simulink model "altitude_contr"  (R2024a)
settings: Solver=FixedStepAuto  StartTime=0.0  StopTime=300  FixedStep=sample_time  RelTol=1e-3
undefined symbols (not defined in the file): A, B, C, D
libraries: slpidlib x1
settings Model: Creator=Lorenzo-Desk  LastModifiedBy=Lorenzo-Desk
settings DataIOCC: ExternalInput=[t,u]

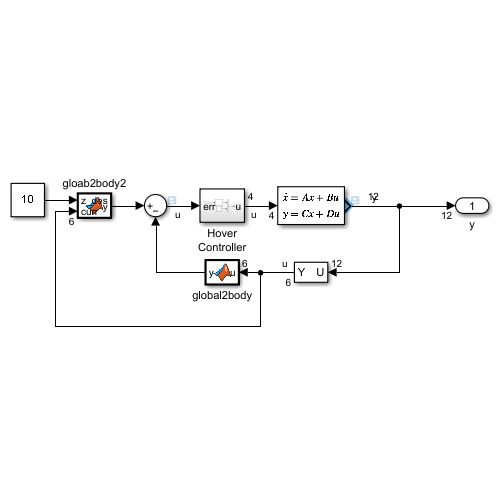
[thumbnail: Simulink's stored preview of the top-level diagram]
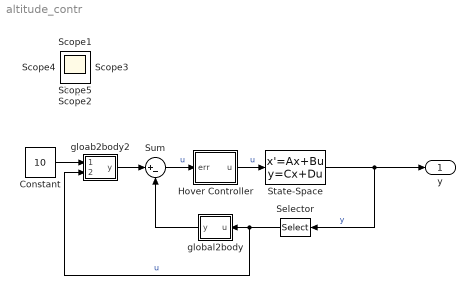
== system altitude_contr ==
  Constant : Constant  Value=10
  Hover Controller : Subsystem
  Selector : Selector  InputPortWidth=12  IndexOptions=Index vector (dialog)  Indices=[1 2 3 7 8 9]  OutputSizes=1
  State-Space : StateSpace  A=A  B=B  C=C  D=D  InitialCondition=0
  Sum : Sum  Inputs=|+-
  gloab2body2 : MATLAB Function  TreatAsAtomicUnit=on
  global2body : MATLAB Function  TreatAsAtomicUnit=on
  y : Outport
  Scope{,1..5} (6 alike) : Scope
  wires:
  State-Space/1 -> Selector/1, y/1  "y"
  Sum/1 -> Hover Controller/1(err)  "u"
  Selector/1 -> gloab2body2/2(curr), global2body/1(u)  "u"
  Constant/1 -> gloab2body2/1(z_des)
  Hover Controller/1(u) -> State-Space/1  "u"
  global2body/1(y) -> Sum/2
  gloab2body2/1(y) -> Sum/1

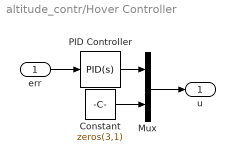
== system altitude_contr/Hover Controller ==
  err : Inport
  Constant : Constant  Value=zeros(3,1)
  Mux : Mux  Inputs=2
  PID Controller : slpidlib/PID Controller  Controller=PID  Form=Parallel  TimeDomain=Continuous-time  UseExternalTs=off  SampleTime=-1  IntegratorMethod=Forward Euler  FilterMethod=Forward Euler  ControllerParametersSource=internal  P=-0.00282534654260682  I=-0.31298101277526e-06  UseKiTs=off  D=-0.14108397495746  UseExternalDerivativeSource=off  N=25.5263564368939  UseFilter=on  TunerSelectOption=Transfer Function Based (PID Tuner App)  InitialConditionSource=internal  InitialConditionForIntegrator=0  InitialConditionForFilter=0  DifferentiatorICPrevScaledInput=0  ExternalReset=none  TrackingMode=off  Kt=1  LimitOutput=on  SatLimitsSource=internal  UpperSaturationLimit=18  LowerSaturationLimit=-18  LinearizeAsGain=on  AntiWindupMode=clamping  Kb=1  LimitIntegrator=on  UpperIntegratorSaturationLimit=20  LowerIntegratorSaturationLimit=-20  POutMin=[]  POutMax=[]  IOutMin=[]  IOutMax=[]  DOutMin=[]  DOutMax=[]  NOutMin=[]  NOutMax=[]  SumOutMin=[]  SumOutMax=[]  SaturationOutMin=[]  SaturationOutMax=[]  PParamMin=[]  PParamMax=[]  IParamMin=[]  IParamMax=[]  DParamMin=[]  DParamMax=[]  NParamMin=[]  NParamMax=[]  KbParamMin=[]  KbParamMax=[]  KtParamMin=[]  KtParamMax=[]  KbOutMin=[]  KbOutMax=[]  KtOutMin=[]  KtOutMax=[]  IntegratorOutMin=[]  IntegratorOutMax=[]  FilterOutMin=[]  FilterOutMax=[]  SumI1OutMin=[]  SumI1OutMax=[]  SumI2OutMin=[]  SumI2OutMax=[]  SumI3OutMin=[]  SumI3OutMax=[]  SumI4OutMin=[]  SumI4OutMax=[]  SumDOutMin=[]  SumDOutMax=[]  DifferentiatorOutMin=[]  DifferentiatorOutMax=[]  FilterDiffOutCoefMin=[]  FilterDiffOutCoefMax=[]  ReciprocalOutMin=[]  ReciprocalOutMax=[]  SumDenOutMin=[]  SumDenOutMax=[]  SumNumOutMin=[]  SumNumOutMax=[]  DivideOutMin=[]  DivideOutMax=[]  UdiffTsProdOutMin=[]  UdiffTsProdOutMax=[]  NTsProdOutMin=[]  NTsProdOutMax=[]  UintegralTsProdOutMin=[]  UintegralTsProdOutMax=[]  UngainTsProdOutMin=[]  UngainTsProdOutMax=[]  ClampingZeroOutDataTypeStr=Inherit: Inherit via back propagation  ClampingZeroOutMin=[]  ClampingZeroOutMax=[]  FilterDenConstantOutDataTypeStr=Inherit: Inherit via back propagation  FilterDenConstantOutMin=[]  FilterDenConstantOutMax=[]  PCopyOutDataTypeStr=Inherit: Inherit via back propagation  PCopyOutMin=[]  PCopyOutMax=[]  NCopyOutDataTypeStr=Inherit: Inherit via back propagation  NCopyOutMin=[]  NCopyOutMax=[]  IntegratorContinuousStateAttributes=''  IntegratorStateMustResolveToSignalObject=off  IntegratorRTWStateStorageClass=Auto  FilterContinuousStateAttributes=''  FilterStateMustResolveToSignalObject=off  FilterRTWStateStorageClass=Auto  ParallelPVariant=InternalParameters  IdealPVariant=Disabled  IVariant=InternalParameters  DVariant=InternalParameters  IntegratorVariant=Continuous  SatVariant=Enabled  AWVariant=ContClampingParallel  PCopyVariant=Disabled  TRVariant=Disabled  FdbkBlocksVariant=Forward  IdealPFdbkVariant=Disabled  SatFdbkVariant=Disabled  DerivativeFilterVariant=ContFilter  NVariant=InternalParameters  NCopyVariant=Disabled  FilterICVariant=InternalICsFilter  IntegratorICVariant=InternalICs  ExternalResetVariant=Disabled  TRSumVariant=Passthrough  SumFdbkVariant=Disabled  SumVariant=Sum_PID  TsampFilterVariant=InternalTs  TsampNgainVariant=Passthrough  TsampIntegralVariant=Disabled_SignalSpec  ExternalSaturationOutDataTypeStr=Inherit: Same as second input  DerivativeSourceVariant=ErrorSignal
  u : Outport
  wires:
  Constant/1 -> Mux/2
  Mux/1 -> u/1
  PID Controller/1 -> Mux/1
  err/1 -> PID Controller/1

== matlab function altitude_contr/global2body ==
  data: u input; y output
function y = fcn(u)
pos = u(1:3); phi = u(4); theta = u(5); psi = u(6);
% define rotation matrix
R_roll = [...
      1, 0, 0;...
      0, cos(phi), -sin(phi);...
      0, sin(phi), cos(phi)];
R_pitch = [...
      cos(theta), 0, sin(theta);...
      0, 1, 0;...
      -sin(theta), 0, cos(theta)];
R_yaw = [...
      cos(psi), -sin(psi), 0;...
      sin(psi), cos(psi), 0;...
      0, 0, 1];  
  
R = R_yaw*R_pitch*R_roll;

pos = pos'*R;
y = pos(3);

== matlab function altitude_contr/gloab2body2 ==
  data: z_des input; y output; curr input
function y = fcn(z_des, curr)
pos = curr(1:3); pos(3) = z_des; phi = curr(4); theta = curr(5); psi = curr(6);
% define rotation matrix
R_roll = [...
      1, 0, 0;...
      0, cos(phi), -sin(phi);...
      0, sin(phi), cos(phi)];
R_pitch = [...
      cos(theta), 0, sin(theta);...
      0, 1, 0;...
      -sin(theta), 0, cos(theta)];
R_yaw = [...
      cos(psi), -sin(psi), 0;...
      sin(psi), cos(psi), 0;...
      0, 0, 1];  
  
R = R_yaw*R_pitch*R_roll;

pos = pos'*R;
y = pos(3);
